simulink model "lvtest_table3"  (Simulink 7.1)
settings: Solver=ode4  StartTime=0.0  StopTime=90  FixedStep=0.01  RelTol=1e-3
values from neighbouring files (symbols this model uses):
  C = abs(d-B)    [fuzzycontrol.m]    (also in lv_demofile6.m = 1450000)
  Ctorque = cq(2:5:102,2:5:182)    [lv_cankaofile.m]    (also in lv_demofile3.m)
  cut_in = 3    [lv_cankaofile.m]    (also in lv_demofile.m; lv_demofile1.m; lv_demofile2.m; lv_demofile3.m)
  cut_out = 25    [lv_cankaofile.m]    (also in lv_demofile.m; lv_demofile1.m; lv_demofile2.m; lv_demofile3.m)
  Jem = 90    [lv_cankaofile.m]    (also in lv_demofile.m = 97.5; lv_demofile1.m = 97.5; lv_demofile2.m = 97.5; lv_demofile3.m = 97.5)
  Jwt = 9e7    (= 90000000)    [lv_cankaofile.m]    (also in lv_demofile.m = 3275300; lv_demofile1.m = 3275300; lv_demofile2.m = 3275300; lv_demofile3.m = 3275300)
  K = 83    [lv_cankaofile.m]    (also in lv_demofile.m; lv_demofile1.m = 75.76; lv_demofile2.m; lv_demofile3.m = 75.76)
  R = 40    [lv_cankaofile.m]    (also in lv_demofile.m = 38.5; lv_demofile1.m = 38.75; lv_demofile2.m = 38.5; lv_demofile3.m = 38.5)
  ro_air = 1.225    [lv_cankaofile.m]    (also in lv_demofile.m = 1.2236; lv_demofile1.m; lv_demofile2.m = 1.2236; lv_demofile3.m)
  roughness = 600    [lv_cankaofile.m]    (also in lv_demofile1.m; lv_demofile3.m; lv_demofile4.m; lv_demofile5.m)
  steptime = 0.01    [lv_cankaofile.m]    (also in lv_demofile1.m; lv_demofile3.m; lv_demofile4.m; lv_demofile5.m)
  Tact = 0    [lv_cankaofile.m]    (also in lv_demofile.m; lv_demofile1.m; lv_demofile2.m; lv_demofile3.m)
  turb_int = 12    [lv_cankaofile.m]    (also in lv_demofile1.m; lv_demofile3.m; lv_demofile4.m; lv_demofile5.m)
undefined symbols (not defined in the file or in its folder): u0
libraries: simulink_extras x1, wt_blockset_v3 x1
settings Model: Creator=xc  LastModifiedBy=lv

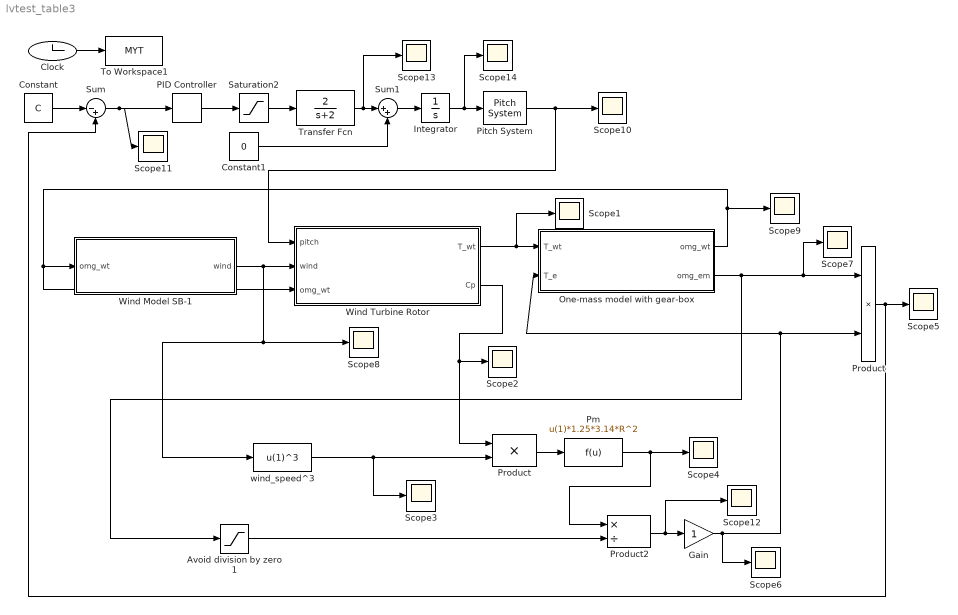
== system lvtest_table3 ==
  Avoid division by zero 1 : Saturate  UpperLimit=1e6  LowerLimit=1e-6  OutDataType=sfix(16)  OutScaling=2^0
  Clock : Clock
      settings: Decimation=10
  Constant : Constant  Value=C  OutDataType=sfix(16)  OutScaling=2^0
  Constant1 : Constant  Value=0  OutDataType=sfix(16)  OutScaling=2^0
  Gain : Gain  ParameterDataType=sfix(16)  ParameterScaling=2^0  OutDataType=sfix(16)  OutScaling=2^0
  Integrator : Integrator
  One-mass model with gear-box : Subsystem  AncestorBlock=wt_blockset_v3/Mechanical Components/One-mass model with gear-box  mask(Simple Gearbox){Jem=Jem, Jwt=Jwt, K=K, init_speed=1.514}
      mask prompts: Jem "Electric machinery - Moment of inertia [kg m2]"; Jwt "Wind turbine rotor - Moment of inertia [kg*m2]"; K "Gearbox ratio"; init_speed "Initial condition [omg_wt (rad/sec)]"
      mask init:
      | J=Jem*K^2+Jwt;
      mask Display: disp('E M\nGear box')
  PID Controller : simulink_extras/Additional Linear/PID Controller  SystemSampleTime=-1  P=5  I=1  D=0
  Pitch System : wt_blockset_v3/Control/WT Controller 2 MW DFIG/Pitch System  SystemSampleTime=-1
  Pm : Fcn  Expr=u(1)*1.25*3.14*R^2
  Product : Product  OutDataType=sfix(16)  OutScaling=2^0  RndMeth=Zero
  "Product " : Product  OutDataType=sfix(16)  OutScaling=2^0  SaturateOnIntegerOverflow=on  OutDataTypeStr=Inherit: Same as first input
  Product2 : Product  Inputs=*/  OutDataType=sfix(16)  OutScaling=2^0  SaturateOnIntegerOverflow=on  OutDataTypeStr=Inherit: Same as first input
  Saturation2 : Saturate  UpperLimit=inf  LowerLimit=1e-6  OutDataType=sfix(16)  OutScaling=2^0
  Scope{1..14} (14 alike) : Scope
      Scope1 settings: YMin=-2.25e+010  YMax=1.5e+010
      Scope10 settings: YMin=-2.25e+010  YMax=1.5e+010  SaveName=ScopeData9
      Scope11 settings: YMin=-2.25e+010  YMax=1.5e+010  SaveName=ScopeData10
      Scope12 settings: SaveName=ScopeData11
      Scope13 settings: YMin=-2.25e+010  YMax=1.5e+010  SaveName=ScopeData12
      Scope14 settings: YMin=-2.25e+010  YMax=1.5e+010  SaveName=ScopeData13
      Scope3 settings: SaveName=ScopeData3
      Scope4 settings: SaveName=ScopeData4
      Scope5 settings: TimeRange=50  YMin=-4000000  YMax=1000000  SaveName=ScopeData6
      Scope6 settings: SaveName=ScopeData5
      Scope7 settings: TimeRange=100  YMin=-9000000  YMax=9000000  SaveName=ScopeData7
      Scope8 settings: YMin=-2.25e+010  YMax=1.5e+010  SaveName=ScopeData17
      Scope9 settings: TimeRange=100  YMin=-9000000  YMax=9000000  SaveName=ScopeData8
  Sum : Sum  Inputs=|-+  OutDataType=sfix(16)  OutScaling=2^0  SaturateOnIntegerOverflow=on
  Sum1 : Sum  Inputs=|++  OutDataType=sfix(16)  OutScaling=2^0  SaturateOnIntegerOverflow=on
  To Workspace1 : ToWorkspace  VariableName=MYT  SampleTime=-1  SaveFormat=Array
  Transfer Fcn : TransferFcn  Numerator=[2]  Denominator=[1 2]
  Wind Model SB-1 : Subsystem  AncestorBlock=wt_blockset_v3/Mechanical Components/Wind Model SB-1  TreatAsAtomicUnit=on  mask(Wind Model using Simulink Band-limited white noise generator){D_rotor=2*R, v_mean=13, roughness=roughness, turb_int=turb_int, T_sample=steptime}
      mask prompts: D_rotor "Rotor diameter [m]"; v_mean "Average wind speed [m/sec]"; roughness "Length scale [m]"; turb_int "Turbulence intensity [%]"; T_sample "Sample time [sec]"
      mask help:
      | Implements a rotor wind model developped by RISOE National Laboratory based on Kaimal spectra. The model takes into account the rotational turbulences and the tower shadow.
      | This model uses the built-in band-limited white noise generator from Simulink with different seeds.
      mask init:
      | r = D_rotor/2;
      | sigma = v_mean*turb_int/100;
      | var = sigma^2;
      | c = roughness/(2*pi*v_mean);
      | d = r/v_mean;
      | trans=sigma*sqrt(roughness/v_mean);
      | random=[256, 894, 31];
      mask Display: disp('Wind\nModel\n(SB-1)')
  Wind Turbine Rotor : Subsystem  AncestorBlock=wt_blockset_beta/Mechanical Components/Wind Turbine Rotor  mask(Aerodynamic model for wind turbine){R=R, ro_air=ro_air, cut_in=cut_in, cut_out=cut_out, Tact=Tact}
      mask prompts: R "Blade radius [m]"; ro_air "Air density [kg m3]"; cut_in "Cut in speed [m/sec]"; cut_out "Cut out speed [m/sec]"; Tact "Time constant for pitch actuator [sec]"
      mask init:
      | %cq_table
      mask Display: plot(20,0,120,200,[45,35,35,45,75,75,45],[85,92,108,115,115,85,85],[55,50,70,65],[115,180,190,115],[55,50,70,65],[85,10,20,85],[75,85],[102,102],[75,85],[98,98],[105,85,85,105],[80,85,115,120])
  wind_speed^3 : Fcn  Expr=u(1)^3
  wires:
  Wind Turbine Rotor/1(T_wt) -> One-mass model with gear-box/1(T_wt), Scope1/1
  Wind Model SB-1/1(wind) -> Scope8/1, wind_speed^3/1, Wind Turbine Rotor/2(wind)
  One-mass model with gear-box/1(omg_wt) -> Wind Turbine Rotor/3(omg_wt), Wind Model SB-1/1(omg_wt), Scope9/1
  One-mass model with gear-box/2(omg_em) -> Avoid division by zero 1/1, Product/1, Scope7/1
  Clock/1 -> To Workspace1/1
  Avoid division by zero 1/1 -> Product2/2
  wind_speed^3/1 -> Scope3/1, "Product "/2
  "Product "/1 -> Pm/1
  Pm/1 -> Scope4/1, Product2/1
  Wind Turbine Rotor/2(Cp) -> Scope2/1, "Product "/1
  Product/1 -> Scope5/1, Sum/2
  Sum/1 -> Scope11/1, PID Controller/1
  Constant/1 -> Sum/1
  Product2/1 -> Gain/1, Scope12/1
  Gain/1 -> Product/2, One-mass model with gear-box/2(T_e), Scope6/1
  PID Controller/1 -> Saturation2/1
  Saturation2/1 -> Transfer Fcn/1
  Pitch System/1 -> Wind Turbine Rotor/1(pitch), Scope10/1
  Transfer Fcn/1 -> Sum1/1, Scope13/1
  Constant1/1 -> Sum1/2
  Sum1/1 -> Integrator/1
  Integrator/1 -> Pitch System/1, Scope14/1

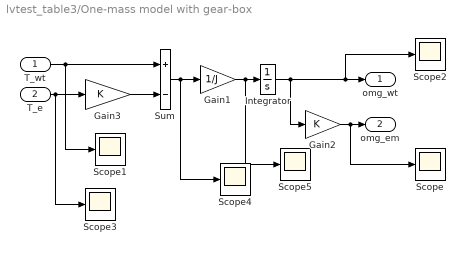
== system lvtest_table3/One-mass model with gear-box ==
  T_wt : Inport  OutDataType=sfix(16)  OutScaling=2^0
  T_e : Inport  Port=2  OutDataType=sfix(16)  OutScaling=2^0
  Gain1 : Gain  Gain=1/J  ParameterDataType=sfix(16)  ParameterScaling=2^0  OutDataType=sfix(16)  OutScaling=2^0  SaturateOnIntegerOverflow=on  OutDataTypeStr=Inherit: Same as input  ParamDataTypeStr=Inherit: Same as input
  Gain2 : Gain  Gain=K  ParameterDataType=sfix(16)  ParameterScaling=2^0  OutDataType=sfix(16)  OutScaling=2^0  SaturateOnIntegerOverflow=on  OutDataTypeStr=Inherit: Same as input  ParamDataTypeStr=Inherit: Same as input
  Gain3 : Gain  Gain=K  ParameterDataType=sfix(16)  ParameterScaling=2^0  OutDataType=sfix(16)  OutScaling=2^0  SaturateOnIntegerOverflow=on  OutDataTypeStr=Inherit: Same as input  ParamDataTypeStr=Inherit: Same as input
  Integrator : Integrator  InitialCondition=init_speed  UpperSaturationLimit=0.95*2*pi*60  LowerSaturationLimit=0
  Scope{,1..5} (6 alike) : Scope
      Scope settings: TimeRange=10  SaveName=ScopeData20
      Scope1 settings: TimeRange=10  SaveName=ScopeData24
      Scope2 settings: YMin=-2.25e+010  YMax=1.5e+010  SaveName=ScopeData21
      Scope3 settings: TimeRange=10  SaveName=ScopeData25
      Scope4 settings: TimeRange=10  SaveName=ScopeData2
      Scope5 settings: TimeRange=10  SaveName=ScopeData22
  Sum : Sum  Inputs=+-  OutDataType=sfix(16)  OutScaling=2^0  SaturateOnIntegerOverflow=on  InputSameDT=on  OutDataTypeStr=Inherit: Same as first input
  omg_wt : Outport  OutDataType=sfix(16)  OutScaling=2^0  InitialOutput=0
  omg_em : Outport  Port=2  OutDataType=sfix(16)  OutScaling=2^0  InitialOutput=0
  wires:
  Gain3/1 -> Sum/2
  Gain2/1 -> omg_em/1, Scope/1
  Integrator/1 -> Gain2/1, omg_wt/1, Scope2/1
  T_wt/1 -> Sum/1, Scope1/1
  T_e/1 -> Gain3/1, Scope3/1
  Sum/1 -> Gain1/1, Scope4/1
  Gain1/1 -> Integrator/1, Scope5/1

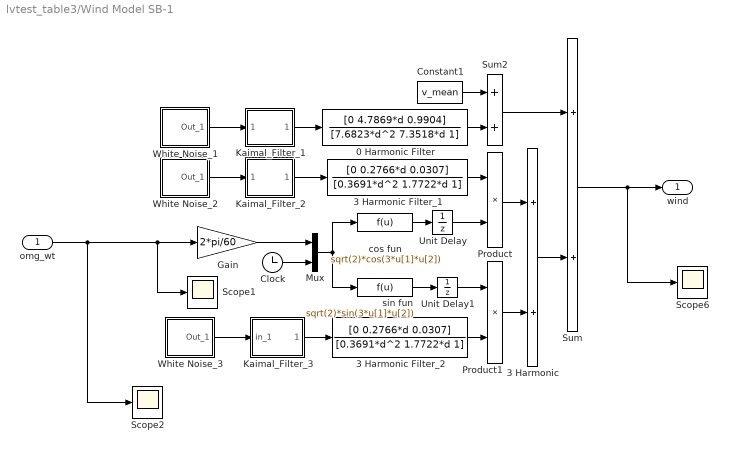
== system lvtest_table3/Wind Model SB-1 ==
  omg_wt : Inport  OutDataType=sfix(16)  OutScaling=2^0
  0 Harmonic Filter : TransferFcn  Numerator=[0 4.7869*d 0.9904]  Denominator=[7.6823*d^2 7.3518*d 1]
  3 Harmonic : Sum  OutDataType=sfix(16)  OutScaling=2^0  SaturateOnIntegerOverflow=on  InputSameDT=on  OutDataTypeStr=Inherit: Same as first input
  3 Harmonic Filter_1 : TransferFcn  Numerator=[0 0.2766*d 0.0307]  Denominator=[0.3691*d^2 1.7722*d 1]
  3 Harmonic Filter_2 : TransferFcn  Numerator=[0 0.2766*d 0.0307]  Denominator=[0.3691*d^2 1.7722*d 1]
  Clock : Clock
  Constant1 : Constant  Value=v_mean  OutDataType=sfix(16)  OutScaling=2^0
  Gain : Gain  Gain=2*pi/60  ParameterDataType=sfix(16)  ParameterScaling=2^0  OutDataType=sfix(16)  OutScaling=2^0  SaturateOnIntegerOverflow=on  OutDataTypeStr=Inherit: Same as input  ParamDataTypeStr=Inherit: Same as input
  Kaimal_Filter_1 : Subsystem
  Kaimal_Filter_2 : Subsystem
  Kaimal_Filter_3 : Subsystem
  Mux : Mux  Inputs=2
  Product : Product  OutDataType=sfix(16)  OutScaling=2^0  SaturateOnIntegerOverflow=on  InputSameDT=on  OutDataTypeStr=Inherit: Same as first input
  Product1 : Product  OutDataType=sfix(16)  OutScaling=2^0  SaturateOnIntegerOverflow=on  InputSameDT=on  OutDataTypeStr=Inherit: Same as first input
  Scope1 : Scope
      settings: YMin=-2.25e+010  YMax=1.5e+010  SaveName=ScopeData22
  Scope2 : Scope
      settings: YMin=-2.25e+010  YMax=1.5e+010  SaveName=ScopeData20
  Scope6 : Scope
      settings: TimeRange=100  YMin=-9e+006  YMax=9e+006  SaveName=ScopeData39
  Sum : Sum  OutDataType=sfix(16)  OutScaling=2^0  SaturateOnIntegerOverflow=on  InputSameDT=on  OutDataTypeStr=Inherit: Same as first input
  Sum2 : Sum  OutDataType=sfix(16)  OutScaling=2^0  SaturateOnIntegerOverflow=on  InputSameDT=on  OutDataTypeStr=Inherit: Same as first input
  Unit Delay : UnitDelay  SampleTime=T_sample
  Unit Delay1 : UnitDelay  SampleTime=T_sample
  White Noise_1 : Subsystem  mask(Continuous White Noise.){Cov=[1], Ts=T_sample, seed=[random(1)]}
      mask prompts: Cov "Noise Power:"; Ts "Sample Time:"
      mask help:
      | White noise for continuous (s-domain) systems.
      | Band-limited using zero-order-hold.
      mask init:
      | r = rand(1,12); r2 = [r(1),r;r,r(12)]; t =[1:13;1:13];
      mask Help: Implemented using white noise into Zero-Order Hold block. The seed and power can be vectors of the same length to produce a vector of white noise sources. For faster simulation, set sample time to the highest value possible but in accordance with the fastest dynamics of system.
      mask Display: plot(t(:),r2(:))
  White Noise_2 : Subsystem  mask(Continuous White Noise.){@1=[1], @2=T_sample, @3=[random(2)]}
      mask prompts: @1 "Noise Power:"; @2 "Sample Time:"; @3 "Seed"
      mask help:
      | White noise for continuous (s-domain) systems.
      | Band-limited using zero-order-hold.
      mask init:
      | Cov = @1; Ts = @2; seed = @3; r = rand(1,12); r2 = [r(1),r;r,r(12)]; t =[1:13;1:13];
      mask Help: Implemented using white noise into Zero-Order Hold block. The seed and power can be vectors of the same length to produce a vector of white noise sources. For faster simulation, set sample time to the highest value possible but in accordance with the fastest dynamics of system.
      mask Display: plot(t(:),r2(:))
  White Noise_3 : Subsystem  mask(Continuous White Noise.){@1=[1], @2=T_sample, @3=[random(3)]}
      mask prompts: @1 "Noise Power:"; @2 "Sample Time:"; @3 "Seed"
      mask help:
      | White noise for continuous (s-domain) systems.
      | Band-limited using zero-order-hold.
      mask init:
      | Cov = @1; Ts = @2; seed = @3; r = rand(1,12); r2 = [r(1),r;r,r(12)]; t =[1:13;1:13];
      mask Help: Implemented using white noise into Zero-Order Hold block. The seed and power can be vectors of the same length to produce a vector of white noise sources. For faster simulation, set sample time to the highest value possible but in accordance with the fastest dynamics of system.
      mask Display: plot(t(:),r2(:))
  cos fun : Fcn  Expr=sqrt(2)*cos(3*u[1]*u[2])
  sin fun : Fcn  Expr=sqrt(2)*sin(3*u[1]*u[2])
  wind : Outport  OutDataType=sfix(16)  OutScaling=2^0  InitialOutput=[u0]
  wires:
  Clock/1 -> Mux/2
  Unit Delay1/1 -> Product1/1
  Unit Delay/1 -> Product/2
  Gain/1 -> Mux/1
  omg_wt/1 -> Gain/1, Scope1/1, Scope2/1
  Mux/1 -> sin fun/1, cos fun/1
  3 Harmonic Filter_1/1 -> Product/1
  White Noise_3/1(Out_1) -> Kaimal_Filter_3/1(in_1)
  White Noise_2/1(Out_1) -> Kaimal_Filter_2/1(in_1)
  White Noise_1/1(Out_1) -> Kaimal_Filter_1/1(in_1)
  Kaimal_Filter_1/1(out_1) -> 0 Harmonic Filter/1
  Sum/1 -> wind/1, Scope6/1
  Constant1/1 -> Sum2/1
  Sum2/1 -> Sum/1
  0 Harmonic Filter/1 -> Sum2/2
  3 Harmonic/1 -> Sum/2
  3 Harmonic Filter_2/1 -> Product1/2
  Product1/1 -> 3 Harmonic/2
  Product/1 -> 3 Harmonic/1
  sin fun/1 -> Unit Delay1/1
  cos fun/1 -> Unit Delay/1
  Kaimal_Filter_3/1(out_1) -> 3 Harmonic Filter_2/1
  Kaimal_Filter_2/1(out_1) -> 3 Harmonic Filter_1/1

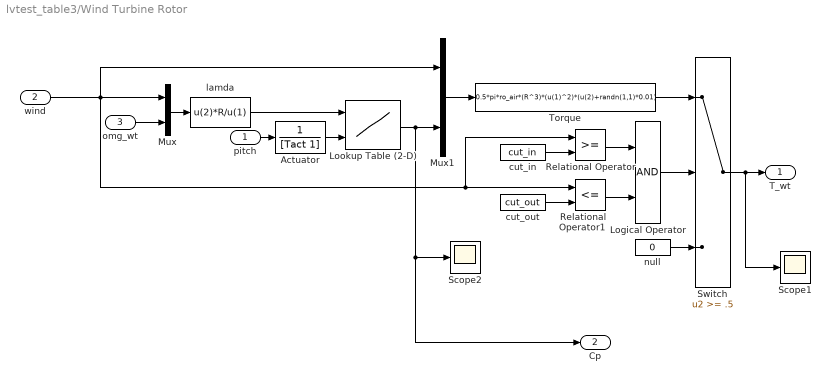
== system lvtest_table3/Wind Turbine Rotor ==
  pitch : Inport  OutDataType=sfix(16)  OutScaling=2^0
  wind : Inport  Port=2  OutDataType=sfix(16)  OutScaling=2^0
  omg_wt : Inport  Port=3  OutDataType=sfix(16)  OutScaling=2^0
  Actuator : TransferFcn  Denominator=[Tact 1]
  Logical Operator : Logic
  Lookup Table (2-D) : Lookup2D  RowIndex=[0:1:20]  ColumnIndex=[-90:5:90]  Table=Ctorque  OutDataType=sfix(16)  OutScaling=2^0
  Mux : Mux  Inputs=2
  Mux1 : Mux  Inputs=2
  Relational Operator : RelationalOperator  InputSameDT=on
  Relational Operator1 : RelationalOperator  Operator=<=  InputSameDT=on
  Scope1 : Scope
      settings: TimeRange=20  YMin=-1500000  YMax=1500000  SaveName=ScopeData19
  Scope2 : Scope
      settings: TimeRange=20  YMin=0.0666  YMax=0.0685  SaveName=ScopeData35
  Switch : Switch  Threshold=.5  SaturateOnIntegerOverflow=on  InputSameDT=on
  Torque : Fcn  Expr=0.5*pi*ro_air*(R^3)*(u(1)^2)*(u(2)+randn(1,1)*0.01)
  cut_in : Constant  Value=cut_in  OutDataType=sfix(16)  OutScaling=2^0
  cut_out : Constant  Value=cut_out  OutDataType=sfix(16)  OutScaling=2^0
  lamda : Fcn  Expr=u(2)*R/u(1)
  null : Constant  Value=0  OutDataType=sfix(16)  OutScaling=2^0
  T_wt : Outport
  Cp : Outport  Port=2
  wires:
  Actuator/1 -> Lookup Table (2-D)/2
  Mux/1 -> lamda/1
  Mux1/1 -> Torque/1
  omg_wt/1 -> Mux/2
  cut_in/1 -> Relational Operator/2
  cut_out/1 -> Relational Operator1/2
  Relational Operator1/1 -> Logical Operator/2
  Relational Operator/1 -> Logical Operator/1
  Switch/1 -> T_wt/1, Scope1/1
  Torque/1 -> Switch/1
  null/1 -> Switch/3
  Logical Operator/1 -> Switch/2
  wind/1 -> Mux/1, Relational Operator/1, Relational Operator1/1, Mux1/1
  Lookup Table (2-D)/1 -> Mux1/2, Scope2/1, Cp/1
  lamda/1 -> Lookup Table (2-D)/1
  pitch/1 -> Actuator/1

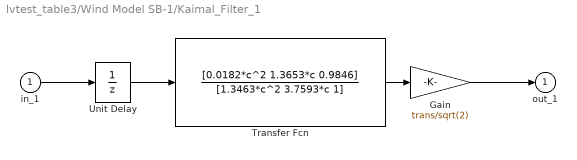
== system lvtest_table3/Wind Model SB-1/Kaimal_Filter_1 ==
  in_1 : Inport  OutDataType=sfix(16)  OutScaling=2^0
  Gain : Gain  Gain=trans/sqrt(2)  ParameterDataType=sfix(16)  ParameterScaling=2^0  OutDataType=sfix(16)  OutScaling=2^0  SaturateOnIntegerOverflow=on  OutDataTypeStr=Inherit: Same as input  ParamDataTypeStr=Inherit: Same as input
  Transfer Fcn : TransferFcn  Numerator=[0.0182*c^2 1.3653*c 0.9846]  Denominator=[1.3463*c^2 3.7593*c 1]
  Unit Delay : UnitDelay  SampleTime=T_sample
  out_1 : Outport  OutDataType=sfix(16)  OutScaling=2^0
  wires:
  Transfer Fcn/1 -> Gain/1
  in_1/1 -> Unit Delay/1
  Gain/1 -> out_1/1
  Unit Delay/1 -> Transfer Fcn/1

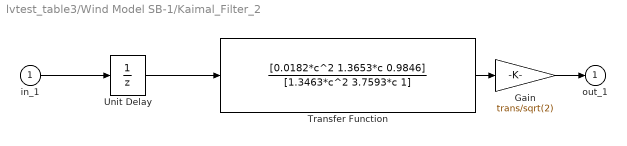
== system lvtest_table3/Wind Model SB-1/Kaimal_Filter_2 ==
  in_1 : Inport  OutDataType=sfix(16)  OutScaling=2^0
  Gain : Gain  Gain=trans/sqrt(2)  ParameterDataType=sfix(16)  ParameterScaling=2^0  OutDataType=sfix(16)  OutScaling=2^0  SaturateOnIntegerOverflow=on  OutDataTypeStr=Inherit: Same as input  ParamDataTypeStr=Inherit: Same as input
  Transfer Function : TransferFcn  Numerator=[0.0182*c^2 1.3653*c 0.9846]  Denominator=[1.3463*c^2 3.7593*c 1]
  Unit Delay : UnitDelay  SampleTime=T_sample
  out_1 : Outport  OutDataType=sfix(16)  OutScaling=2^0
  wires:
  Transfer Function/1 -> Gain/1
  in_1/1 -> Unit Delay/1
  Gain/1 -> out_1/1
  Unit Delay/1 -> Transfer Function/1

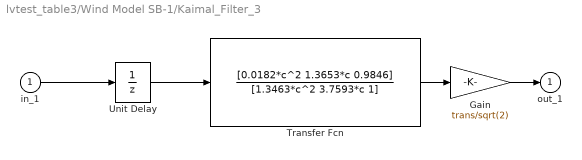
== system lvtest_table3/Wind Model SB-1/Kaimal_Filter_3 ==
  in_1 : Inport  OutDataType=sfix(16)  OutScaling=2^0
  Gain : Gain  Gain=trans/sqrt(2)  ParameterDataType=sfix(16)  ParameterScaling=2^0  OutDataType=sfix(16)  OutScaling=2^0  SaturateOnIntegerOverflow=on  OutDataTypeStr=Inherit: Same as input  ParamDataTypeStr=Inherit: Same as input
  Transfer Fcn : TransferFcn  Numerator=[0.0182*c^2 1.3653*c 0.9846]  Denominator=[1.3463*c^2 3.7593*c 1]
  Unit Delay : UnitDelay  SampleTime=T_sample
  out_1 : Outport  OutDataType=sfix(16)  OutScaling=2^0
  wires:
  Transfer Fcn/1 -> Gain/1
  in_1/1 -> Unit Delay/1
  Gain/1 -> out_1/1
  Unit Delay/1 -> Transfer Fcn/1

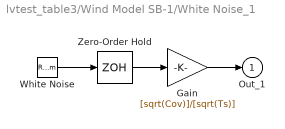
== system lvtest_table3/Wind Model SB-1/White Noise_1 ==
  Gain : Gain  Gain=[sqrt(Cov)]/[sqrt(Ts)]  ParameterDataType=sfix(16)  ParameterScaling=2^0  OutDataType=sfix(16)  OutScaling=2^0  SaturateOnIntegerOverflow=on  OutDataTypeStr=Inherit: Same as input  ParamDataTypeStr=Inherit: Same as input
  White Noise : RandomNumber  Seed=seed  SampleTime=Ts
  Zero-Order Hold : ZeroOrderHold  SampleTime=Ts
  Out_1 : Outport  OutDataType=sfix(16)  OutScaling=2^0
  wires:
  Zero-Order Hold/1 -> Gain/1
  Gain/1 -> Out_1/1
  White Noise/1 -> Zero-Order Hold/1

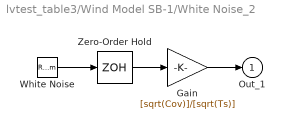
== system lvtest_table3/Wind Model SB-1/White Noise_2 ==
  Gain : Gain  Gain=[sqrt(Cov)]/[sqrt(Ts)]  ParameterDataType=sfix(16)  ParameterScaling=2^0  OutDataType=sfix(16)  OutScaling=2^0  SaturateOnIntegerOverflow=on  OutDataTypeStr=Inherit: Same as input  ParamDataTypeStr=Inherit: Same as input
  White Noise : RandomNumber  Seed=seed  SampleTime=Ts
  Zero-Order Hold : ZeroOrderHold  SampleTime=Ts
  Out_1 : Outport  OutDataType=sfix(16)  OutScaling=2^0
  wires:
  Zero-Order Hold/1 -> Gain/1
  Gain/1 -> Out_1/1
  White Noise/1 -> Zero-Order Hold/1

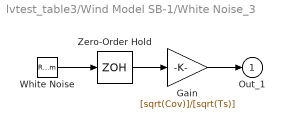
== system lvtest_table3/Wind Model SB-1/White Noise_3 ==
  Gain : Gain  Gain=[sqrt(Cov)]/[sqrt(Ts)]  ParameterDataType=sfix(16)  ParameterScaling=2^0  OutDataType=sfix(16)  OutScaling=2^0  SaturateOnIntegerOverflow=on  OutDataTypeStr=Inherit: Same as input  ParamDataTypeStr=Inherit: Same as input
  White Noise : RandomNumber  Seed=seed  SampleTime=Ts
  Zero-Order Hold : ZeroOrderHold  SampleTime=Ts
  Out_1 : Outport  OutDataType=sfix(16)  OutScaling=2^0
  wires:
  Zero-Order Hold/1 -> Gain/1
  Gain/1 -> Out_1/1
  White Noise/1 -> Zero-Order Hold/1
